simulink model "two_generator_droop"  (R2014a)
settings: Solver=ode23tb  StartTime=0.0  StopTime=5  MaxStep=1/60  RelTol=1e-4
PreLoadFcn:
  | d1 = 0.05;
  | d2 = 0.04;
  | Ts= 1e-4;
libraries: powerlib x6, simulink x4, powerlib_meascontrol x2
settings Model: Creator=gdudgeon  LastModifiedBy=cosorio
settings DataIOCC: SaveOutput=off  SaveTime=off
settings OptimizationCC: ExpressionDepthLimit=2147483647
settings DebuggingCC: UnderspecifiedInitializationDetection=Classic  SolverPrmCheckMsg=none  FcnCallInpInsideContextMsg=UseLocalSettings  StateNameClashWarn=warning
settings GRTTargetCC: CombineOutputUpdateFcns=off  GRTInterface=on

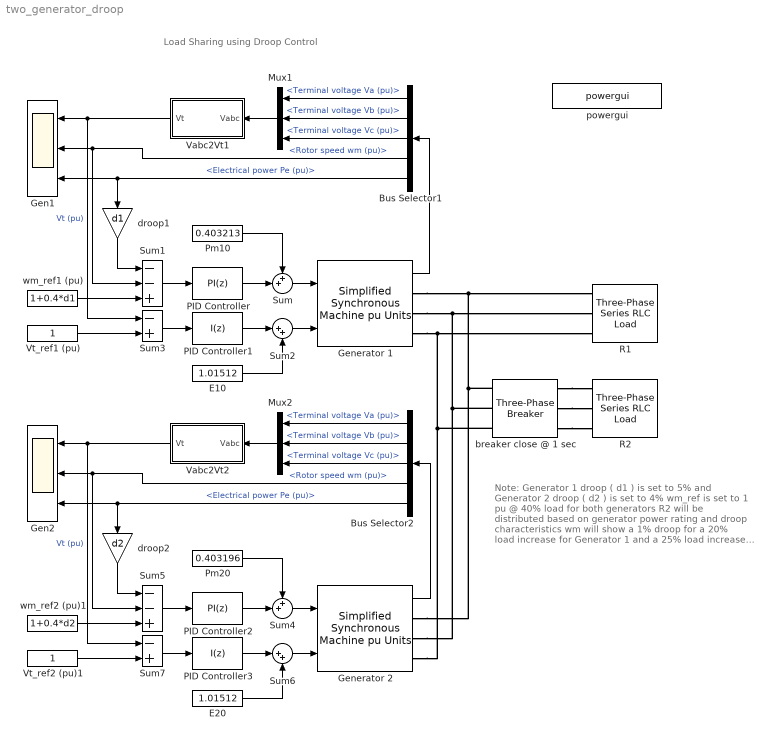
== system two_generator_droop ==
  note: Note:
      | Generator 1 droop ( d1 ) is set to 5% and Generator 2 droop ( d2 ) is set to 4%
      | wm_ref is set to 1 pu @ 40% load for both generators
      | R2 will be distributed based on generator power rating and droop characteristics
      | wm will show a 1% droop for a 20% load increase for Generator 1 and a 25% load increase for Generator 2
  note: Load Sharing using Droop Control
  Bus Selector1 : BusSelector  OutputSignals=Terminal voltage Va (pu),Terminal voltage Vb (pu),Terminal voltage Vc (pu),Rotor speed wm (pu),Electrical power Pe (pu)
  Bus Selector2 : BusSelector  OutputSignals=Terminal voltage Va (pu),Terminal voltage Vb (pu),Terminal voltage Vc (pu),Rotor speed wm (pu),Electrical power Pe (pu)
  E10 : Constant  Value=1.01512
  E20 : Constant  Value=1.01512
  Gen1 : Scope  NumInputPorts=3
      settings: YMin=0~0.97~0.3  YMax=1.5~1.01~0.7  SaveName=Gen1
  Gen2 : Scope  NumInputPorts=3
      settings: YMin=0~0.97~0.3  YMax=1.5~1.01~0.7  SaveName=Gen2
  Generator 1 : powerlib/Machines/Simplified Synchronous Machine pu Units  ConnectionType=3-wire Y  MechanicalLoad=Mechanical power Pm  MeasurementBus=off  NominalParameters=[5e6 6600 60]  Mechanical=[3.7 0 20]  InternalRL="[0.02  0.3]"  InitialConditions=[0 6.78919 0.400013 0.400013 0.400013 0 -120 120]  Units=0  LoadFlowParameters=[2 2000000 0 0 0]  TsPowergui=0  TsBlock=-1  BusType=PV  Pref=0  Qref=0  Qmin=-inf  Qmax=+inf  PLF=0  QLF=0
      settings: AttributesFormatString=%<NominalParameters>
  Generator 2 : powerlib/Machines/Simplified Synchronous Machine pu Units  ConnectionType=3-wire Y  MechanicalLoad=Mechanical power Pm  MeasurementBus=off  NominalParameters=[5e6 6600 60]  Mechanical=[3.7 0 20]  InternalRL="[0.02  0.3]"  InitialConditions=[0 6.78891 0.399996 0.399996 0.399996 0 -120 120]  Units=0  LoadFlowParameters=[2 2000000 0 0 0]  TsPowergui=0  TsBlock=-1  BusType=PV  Pref=0  Qref=0  Qmin=-inf  Qmax=+inf  PLF=0  QLF=0
      settings: AttributesFormatString=%<NominalParameters>
  Mux1 : Mux  Inputs=3
  Mux2 : Mux  Inputs=3
  PID Controller : simulink/Continuous/PID Controller  Controller=PI  TimeDomain=Discrete-time  SampleTime=Ts  IntegratorMethod=Forward Euler  FilterMethod=Forward Euler  Form=Parallel  P=25  I=50  D=0  N=100  InitialConditionSource=internal  InitialConditionForIntegrator=0  InitialConditionForFilter=0  ExternalReset=none  LimitOutput=off  UpperSaturationLimit=inf  LowerSaturationLimit=-inf  LinearizeAsGain=on  AntiWindupMode=none  Kb=1  TrackingMode=off  Kt=1  PParamMin=[]  PParamMax=[]  IParamMin=[]  IParamMax=[]  DParamMin=[]  DParamMax=[]  NParamMin=[]  NParamMax=[]  KbParamMin=[]  KbParamMax=[]  KtParamMin=[]  KtParamMax=[]  POutMin=[]  POutMax=[]  IOutMin=[]  IOutMax=[]  DOutMin=[]  DOutMax=[]  NOutMin=[]  NOutMax=[]  KbOutMin=[]  KbOutMax=[]  KtOutMin=[]  KtOutMax=[]  IntegratorOutMin=[]  IntegratorOutMax=[]  FilterOutMin=[]  FilterOutMax=[]  SumOutMin=[]  SumOutMax=[]  SumI1OutMin=[]  SumI1OutMax=[]  SumI2OutMin=[]  SumI2OutMax=[]  SumI3OutMin=[]  SumI3OutMax=[]  SumDOutMin=[]  SumDOutMax=[]  SaturationOutMin=[]  SaturationOutMax=[]  IntegratorContinuousStateAttributes=''  IntegratorStateMustResolveToSignalObject=off  IntegratorRTWStateStorageClass=Auto  FilterContinuousStateAttributes=''  FilterStateMustResolveToSignalObject=off  FilterRTWStateStorageClass=Auto
  PID Controller1 : simulink/Continuous/PID Controller  Controller=I  TimeDomain=Discrete-time  SampleTime=Ts  IntegratorMethod=Forward Euler  FilterMethod=Forward Euler  Form=Parallel  P=0  I=30  D=0  N=100  InitialConditionSource=internal  InitialConditionForIntegrator=0  InitialConditionForFilter=0  ExternalReset=none  LimitOutput=off  UpperSaturationLimit=inf  LowerSaturationLimit=-inf  LinearizeAsGain=on  AntiWindupMode=none  Kb=1  TrackingMode=off  Kt=1  PParamMin=[]  PParamMax=[]  IParamMin=[]  IParamMax=[]  DParamMin=[]  DParamMax=[]  NParamMin=[]  NParamMax=[]  KbParamMin=[]  KbParamMax=[]  KtParamMin=[]  KtParamMax=[]  POutMin=[]  POutMax=[]  IOutMin=[]  IOutMax=[]  DOutMin=[]  DOutMax=[]  NOutMin=[]  NOutMax=[]  KbOutMin=[]  KbOutMax=[]  KtOutMin=[]  KtOutMax=[]  IntegratorOutMin=[]  IntegratorOutMax=[]  FilterOutMin=[]  FilterOutMax=[]  SumOutMin=[]  SumOutMax=[]  SumI1OutMin=[]  SumI1OutMax=[]  SumI2OutMin=[]  SumI2OutMax=[]  SumI3OutMin=[]  SumI3OutMax=[]  SumDOutMin=[]  SumDOutMax=[]  SaturationOutMin=[]  SaturationOutMax=[]  IntegratorContinuousStateAttributes=''  IntegratorStateMustResolveToSignalObject=off  IntegratorRTWStateStorageClass=Auto  FilterContinuousStateAttributes=''  FilterStateMustResolveToSignalObject=off  FilterRTWStateStorageClass=Auto
  PID Controller2 : simulink/Continuous/PID Controller  Controller=PI  TimeDomain=Discrete-time  SampleTime=Ts  IntegratorMethod=Forward Euler  FilterMethod=Forward Euler  Form=Parallel  P=25  I=50  D=0  N=100  InitialConditionSource=internal  InitialConditionForIntegrator=0  InitialConditionForFilter=0  ExternalReset=none  LimitOutput=off  UpperSaturationLimit=inf  LowerSaturationLimit=-inf  LinearizeAsGain=on  AntiWindupMode=none  Kb=1  TrackingMode=off  Kt=1  PParamMin=[]  PParamMax=[]  IParamMin=[]  IParamMax=[]  DParamMin=[]  DParamMax=[]  NParamMin=[]  NParamMax=[]  KbParamMin=[]  KbParamMax=[]  KtParamMin=[]  KtParamMax=[]  POutMin=[]  POutMax=[]  IOutMin=[]  IOutMax=[]  DOutMin=[]  DOutMax=[]  NOutMin=[]  NOutMax=[]  KbOutMin=[]  KbOutMax=[]  KtOutMin=[]  KtOutMax=[]  IntegratorOutMin=[]  IntegratorOutMax=[]  FilterOutMin=[]  FilterOutMax=[]  SumOutMin=[]  SumOutMax=[]  SumI1OutMin=[]  SumI1OutMax=[]  SumI2OutMin=[]  SumI2OutMax=[]  SumI3OutMin=[]  SumI3OutMax=[]  SumDOutMin=[]  SumDOutMax=[]  SaturationOutMin=[]  SaturationOutMax=[]  IntegratorContinuousStateAttributes=''  IntegratorStateMustResolveToSignalObject=off  IntegratorRTWStateStorageClass=Auto  FilterContinuousStateAttributes=''  FilterStateMustResolveToSignalObject=off  FilterRTWStateStorageClass=Auto
  PID Controller3 : simulink/Continuous/PID Controller  Controller=I  TimeDomain=Discrete-time  SampleTime=Ts  IntegratorMethod=Forward Euler  FilterMethod=Forward Euler  Form=Parallel  P=0  I=30  D=0  N=100  InitialConditionSource=internal  InitialConditionForIntegrator=0  InitialConditionForFilter=0  ExternalReset=none  LimitOutput=off  UpperSaturationLimit=inf  LowerSaturationLimit=-inf  LinearizeAsGain=on  AntiWindupMode=none  Kb=1  TrackingMode=off  Kt=1  PParamMin=[]  PParamMax=[]  IParamMin=[]  IParamMax=[]  DParamMin=[]  DParamMax=[]  NParamMin=[]  NParamMax=[]  KbParamMin=[]  KbParamMax=[]  KtParamMin=[]  KtParamMax=[]  POutMin=[]  POutMax=[]  IOutMin=[]  IOutMax=[]  DOutMin=[]  DOutMax=[]  NOutMin=[]  NOutMax=[]  KbOutMin=[]  KbOutMax=[]  KtOutMin=[]  KtOutMax=[]  IntegratorOutMin=[]  IntegratorOutMax=[]  FilterOutMin=[]  FilterOutMax=[]  SumOutMin=[]  SumOutMax=[]  SumI1OutMin=[]  SumI1OutMax=[]  SumI2OutMin=[]  SumI2OutMax=[]  SumI3OutMin=[]  SumI3OutMax=[]  SumDOutMin=[]  SumDOutMax=[]  SaturationOutMin=[]  SaturationOutMax=[]  IntegratorContinuousStateAttributes=''  IntegratorStateMustResolveToSignalObject=off  IntegratorRTWStateStorageClass=Auto  FilterContinuousStateAttributes=''  FilterStateMustResolveToSignalObject=off  FilterRTWStateStorageClass=Auto
  Pm10 : Constant  Value=0.403213
  Pm20 : Constant  Value=0.403196
  R1 : powerlib/Elements/Three-Phase Series RLC Load  LConnTagsString=A|B|C  Configuration=Y (grounded)  NominalVoltage=6600  NominalFrequency=60  ActivePower=4e6  InductivePower=0  CapacitivePower=0  Measurements=None  LoadType=constant Z
      settings: AttributesFormatString=P = %<ActivePower> W
  "R2 " : powerlib/Elements/Three-Phase Series RLC Load  LConnTagsString=A|B|C  Configuration=Y (grounded)  NominalVoltage=6600  NominalFrequency=60  ActivePower=2.25e6  InductivePower=0  CapacitivePower=0  Measurements=None  LoadType=constant Z
      settings: AttributesFormatString=P = %<ActivePower> W
  Sum : Sum  Inputs=++|
  Sum1 : Sum  Inputs=--+
  Sum2 : Sum  Inputs=|++
  Sum3 : Sum  Inputs=-+
  Sum4 : Sum  Inputs=++|
  Sum5 : Sum  Inputs=--+
  Sum6 : Sum  Inputs=|++
  Sum7 : Sum  Inputs=-+
  Vabc2Vt1 : Subsystem
  Vabc2Vt2 : Subsystem
  Vt_ref1 (pu) : Constant
  Vt_ref2 (pu)1 : Constant
  breaker close @ 1 sec : powerlib/Elements/Three-Phase Breaker  InitialState=open  SwitchA=on  SwitchB=on  SwitchC=on  SwitchTimes=1  External=off  BreakerResistance=1e-5  SnubberResistance=1e6  SnubberCapacitance=inf  Measurements=None
  droop1 : Gain  Gain=d1
  droop2 : Gain  Gain=d2
  powergui : powerlib/powergui  SimulationMode=Discrete  SolverType=Tustin  SampleTime=1e-4  frequency=60  SPID=off  DisableSnubberDevices=off  DisableRonSwitches=off  DisableVfSwitches=off  SwTol=0  Interpol=off  DisplayEquations=off  Ts=0  methode=off  frequencyindice=60  Pbase=100e6  ErrMax=1e-4  Iterations=50  UnitsV=kV  UnitsW=MW  FunctionMessages=off  echomessages=off  HookPort=off  EnableUseOfTLC=off  x0status=blocks  RestoreLinks=warning  ResistiveCurrentMeasurement=off  Frange=[0:2:500]  Ylog=off  Xlog=on  ShowGrid=off  save=off  variable=ZData  structure=0  ZoomFFT=on  StartTime=0.0  cycles=1  DisplayStyle=1  fundamental=60  FreqAxis=off  MaxFrequency=1000  frequencyindicesteady=1  RmsSteady=1  display=off
  wm_ref1 (pu) : Constant  Value=1+0.4*d1
  wm_ref2 (pu)1 : Constant  Value=1+0.4*d2
  wires:
  Generator 1/1 -> Bus Selector1/1
  Sum1/1 -> PID Controller/1
  Sum3/1 -> PID Controller1/1
  wm_ref1 (pu)/1 -> Sum1/3
  Bus Selector1/5 -> Gen1/3, droop1/1  "<Electrical power Pe (pu)>"
  droop1/1 -> Sum1/1
  PID Controller1/1 -> Sum2/1
  PID Controller/1 -> Sum/2
  E10/1 -> Sum2/2
  Sum2/1 -> Generator 1/2
  Pm10/1 -> Sum/1
  Sum/1 -> Generator 1/1
  Bus Selector1/4 -> Sum1/2, Gen1/2  "<Rotor speed wm (pu)>"
  Bus Selector1/3 -> Mux1/3  "<Terminal voltage Vc (pu)>"
  Bus Selector1/2 -> Mux1/2  "<Terminal voltage Vb (pu)>"
  Bus Selector1/1 -> Mux1/1  "<Terminal voltage Va (pu)>"
  Mux1/1 -> Vabc2Vt1/1(Vabc)
  Vt_ref1 (pu)/1 -> Sum3/2
  Vabc2Vt1/1(Vt) -> Sum3/1, Gen1/1  "Vt (pu)"
  Generator 2/1 -> Bus Selector2/1
  Sum5/1 -> PID Controller2/1
  Sum7/1 -> PID Controller3/1
  wm_ref2 (pu)1/1 -> Sum5/3
  Bus Selector2/5 -> Gen2/3, droop2/1  "<Electrical power Pe (pu)>"
  droop2/1 -> Sum5/1
  PID Controller3/1 -> Sum6/1
  PID Controller2/1 -> Sum4/2
  E20/1 -> Sum6/2
  Sum6/1 -> Generator 2/2
  Pm20/1 -> Sum4/1
  Sum4/1 -> Generator 2/1
  Bus Selector2/4 -> Gen2/2, Sum5/2  "<Rotor speed wm (pu)>"
  Bus Selector2/3 -> Mux2/3  "<Terminal voltage Vc (pu)>"
  Bus Selector2/2 -> Mux2/2  "<Terminal voltage Vb (pu)>"
  Bus Selector2/1 -> Mux2/1  "<Terminal voltage Va (pu)>"
  Mux2/1 -> Vabc2Vt2/1(Vabc)
  Vt_ref2 (pu)1/1 -> Sum7/2
  Vabc2Vt2/1(Vt) -> Gen2/1, Sum7/1  "Vt (pu)"
  connections:
  breaker close @ 1 sec/LConn1 -- Generator 2/RConn1 -- Generator 1/RConn1 -- R1/LConn1
  breaker close @ 1 sec/LConn2 -- Generator 2/RConn2 -- Generator 1/RConn2 -- R1/LConn2
  breaker close @ 1 sec/LConn3 -- Generator 2/RConn3 -- R1/LConn3 -- Generator 1/RConn3
  breaker close @ 1 sec/RConn1 -- "R2 "/LConn1
  breaker close @ 1 sec/RConn2 -- "R2 "/LConn2
  breaker close @ 1 sec/RConn3 -- "R2 "/LConn3

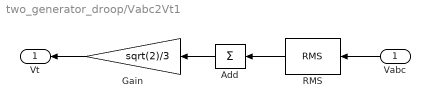
== system two_generator_droop/Vabc2Vt1 ==
  Vabc : Inport
  Add : Sum  Inputs=+
  Gain : Gain  Gain=sqrt(2)/3
  RMS : powerlib_meascontrol/Measurements/RMS  TrueRMS=on  Freq=60  RMSInit=1/sqrt(2)  Ts=Ts
  Vt : Outport
  wires:
  RMS/1 -> Add/1
  Gain/1 -> Vt/1
  Add/1 -> Gain/1
  Vabc/1 -> RMS/1

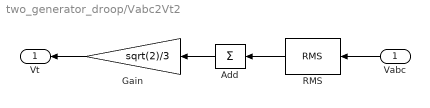
== system two_generator_droop/Vabc2Vt2 ==
  Vabc : Inport
  Add : Sum  Inputs=+
  Gain : Gain  Gain=sqrt(2)/3
  RMS : powerlib_meascontrol/Measurements/RMS  TrueRMS=on  Freq=60  RMSInit=1/sqrt(2)  Ts=Ts
  Vt : Outport
  wires:
  Vabc/1 -> RMS/1
  Add/1 -> Gain/1
  Gain/1 -> Vt/1
  RMS/1 -> Add/1
